simulink model "BLDCFramework"  (R2026a)
settings: Solver=FixedStepAuto  StopTime=4  FixedStep=6.25e-5
undefined symbols (not defined in the file): BldcControl_Params, BldcRuntime_Init
settings Model: DataDictionary=BldcData.sldd  Creator=k  LastModifiedBy=k
settings OptimizationCC: UseDivisionForNetSlopeComputation=on  GainParamInheritBuiltInType=on  UseFloatMulNetSlope=on  InlineInvariantSignals=on  NoFixptDivByZeroProtection=on  EfficientFloat2IntCast=on  LifeSpan=1
settings RTWCC: SystemTargetFile=ert.tlc  GenerateReport=on  Toolchain=MinGW64 | gmake (64-bit Windows)  IncludeHyperlinkInReport=on  GenerateTraceInfo=on  GenerateTraceReport=on  GenerateTraceReportSl=on  GenerateTraceReportSf=on  GenerateTraceReportEml=on  GenerateCodeMetricsReport=on  Description=Embedded Coder
settings ERTTargetCC: GenerateSampleERTMain=on  IncludeMdlTerminateFcn=off  CombineSignalStateStructs=on  SupportComplex=off  SupportContinuousTime=on  SupportNonInlinedSFcns=on

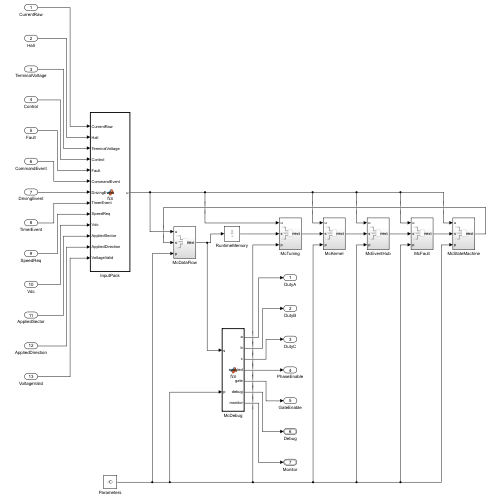
[thumbnail: Simulink's stored preview of the top-level diagram]
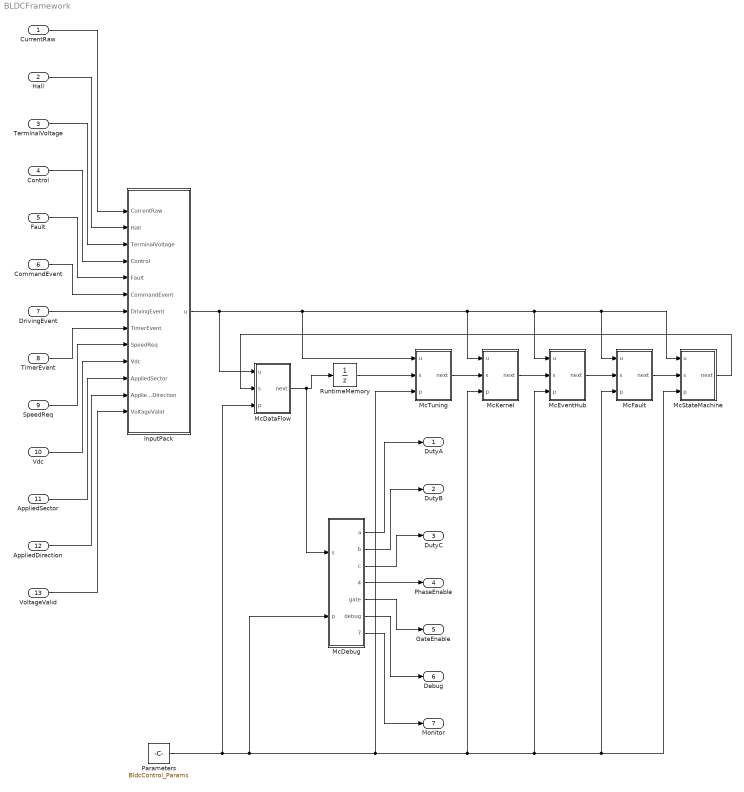
== system BLDCFramework ==
  CurrentRaw : Inport  OutDataTypeStr=uint16  PortDimensions=3  SampleTime=6.25e-5
  Hall : Inport  Port=2  OutDataTypeStr=uint8  PortDimensions=1  SampleTime=6.25e-5
  TerminalVoltage : Inport  Port=3  OutDataTypeStr=single  PortDimensions=3  SampleTime=6.25e-5
  Control : Inport  Port=4  OutDataTypeStr=uint8  PortDimensions=1  SampleTime=6.25e-5
  Fault : Inport  Port=5  OutDataTypeStr=boolean  PortDimensions=1  SampleTime=6.25e-5
  CommandEvent : Inport  Port=6  OutDataTypeStr=boolean  PortDimensions=1  SampleTime=6.25e-5
  DrivingEvent : Inport  Port=7  OutDataTypeStr=boolean  PortDimensions=1  SampleTime=6.25e-5
  TimerEvent : Inport  Port=8  OutDataTypeStr=boolean  PortDimensions=1  SampleTime=6.25e-5
  SpeedReq : Inport  Port=9  OutDataTypeStr=single  PortDimensions=1  SampleTime=6.25e-5
  Vdc : Inport  Port=10  OutDataTypeStr=single  PortDimensions=1  SampleTime=6.25e-5
  AppliedSector : Inport  Port=11  OutDataTypeStr=uint8  PortDimensions=1  SampleTime=6.25e-5
  AppliedDirection : Inport  Port=12  OutDataTypeStr=int8  PortDimensions=1  SampleTime=6.25e-5
  VoltageValid : Inport  Port=13  OutDataTypeStr=boolean  PortDimensions=1  SampleTime=6.25e-5
  InputPack : MATLAB Function  TreatAsAtomicUnit=on
  McDataFlow : Subsystem
  McDebug : MATLAB Function  TreatAsAtomicUnit=on
  McEventHub : Subsystem
  McFault : Subsystem
  McKernel : Subsystem
  McStateMachine : Subsystem
  McTuning : Subsystem
  Parameters : Constant  Value=BldcControl_Params  OutDataTypeStr=Bus: tBldcParams
  RuntimeMemory : UnitDelay  InitialCondition=BldcRuntime_Init  SampleTime=6.25e-5
  DutyA : Outport  OutDataTypeStr=uint16  PortDimensions=1
  DutyB : Outport  Port=2  OutDataTypeStr=uint16  PortDimensions=1
  DutyC : Outport  Port=3  OutDataTypeStr=uint16  PortDimensions=1
  PhaseEnable : Outport  Port=4  OutDataTypeStr=boolean  PortDimensions=3
  GateEnable : Outport  Port=5  OutDataTypeStr=boolean  PortDimensions=1
  Debug : Outport  Port=6  OutDataTypeStr=Bus: tBldcDebug  PortDimensions=1
  Monitor : Outport  Port=7  OutDataTypeStr=Bus: tBldcMonitor  PortDimensions=1
  wires:
  McDebug/7(monitor) -> Monitor/1
  McDebug/6(debug) -> Debug/1
  McDebug/5(gate) -> GateEnable/1
  McDebug/4(enabled) -> PhaseEnable/1
  McDebug/3(c) -> DutyC/1
  McDebug/2(b) -> DutyB/1
  McDebug/1(a) -> DutyA/1
  McDataFlow/1(next) -> McDebug/1(s), RuntimeMemory/1
  McStateMachine/1(next) -> McDataFlow/2(s)
  McFault/1(next) -> McStateMachine/2(s)
  McEventHub/1(next) -> McFault/2(s)
  McKernel/1(next) -> McEventHub/2(s)
  McTuning/1(next) -> McKernel/2(s)
  Parameters/1 -> McStateMachine/3(p), McFault/3(p), McEventHub/3(p), McKernel/3(p), McTuning/3(p), McDebug/2(p), McDataFlow/3(p)
  RuntimeMemory/1 -> McTuning/2(s)
  InputPack/1(u) -> McFault/1(u), McStateMachine/1(u), McEventHub/1(u), McKernel/1(u), McTuning/1(u), McDataFlow/1(u)
  VoltageValid/1 -> InputPack/13(VoltageValid)
  AppliedDirection/1 -> InputPack/12(AppliedDirection)
  AppliedSector/1 -> InputPack/11(AppliedSector)
  Vdc/1 -> InputPack/10(Vdc)
  SpeedReq/1 -> InputPack/9(SpeedReq)
  TimerEvent/1 -> InputPack/8(TimerEvent)
  DrivingEvent/1 -> InputPack/7(DrivingEvent)
  CommandEvent/1 -> InputPack/6(CommandEvent)
  Fault/1 -> InputPack/5(Fault)
  Control/1 -> InputPack/4(Control)
  TerminalVoltage/1 -> InputPack/3(TerminalVoltage)
  Hall/1 -> InputPack/2(Hall)
  CurrentRaw/1 -> InputPack/1(CurrentRaw)

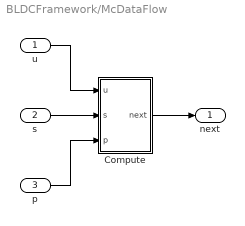
== system BLDCFramework/McDataFlow ==
  u : Inport  OutDataTypeStr=Bus: tBldcInput  PortDimensions=1  SampleTime=6.25e-5
  s : Inport  Port=2  OutDataTypeStr=Bus: tBldcRuntime  PortDimensions=1  SampleTime=6.25e-5
  p : Inport  Port=3  OutDataTypeStr=Bus: tBldcParams  PortDimensions=1  SampleTime=6.25e-5
  Compute : MATLAB Function  TreatAsAtomicUnit=on
  next : Outport  OutDataTypeStr=Bus: tBldcRuntime  PortDimensions=1
  wires:
  Compute/1(next) -> next/1
  p/1 -> Compute/3(p)
  s/1 -> Compute/2(s)
  u/1 -> Compute/1(u)

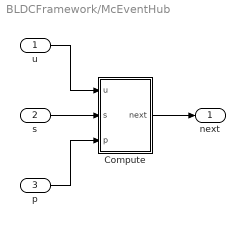
== system BLDCFramework/McEventHub ==
  u : Inport  OutDataTypeStr=Bus: tBldcInput  PortDimensions=1  SampleTime=6.25e-5
  s : Inport  Port=2  OutDataTypeStr=Bus: tBldcRuntime  PortDimensions=1  SampleTime=6.25e-5
  p : Inport  Port=3  OutDataTypeStr=Bus: tBldcParams  PortDimensions=1  SampleTime=6.25e-5
  Compute : MATLAB Function  TreatAsAtomicUnit=on
  next : Outport  OutDataTypeStr=Bus: tBldcRuntime  PortDimensions=1
  wires:
  Compute/1(next) -> next/1
  p/1 -> Compute/3(p)
  s/1 -> Compute/2(s)
  u/1 -> Compute/1(u)

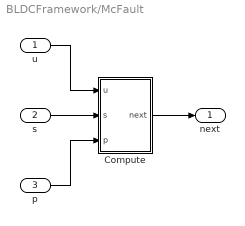
== system BLDCFramework/McFault ==
  u : Inport  OutDataTypeStr=Bus: tBldcInput  PortDimensions=1  SampleTime=6.25e-5
  s : Inport  Port=2  OutDataTypeStr=Bus: tBldcRuntime  PortDimensions=1  SampleTime=6.25e-5
  p : Inport  Port=3  OutDataTypeStr=Bus: tBldcParams  PortDimensions=1  SampleTime=6.25e-5
  Compute : MATLAB Function  TreatAsAtomicUnit=on
  next : Outport  OutDataTypeStr=Bus: tBldcRuntime  PortDimensions=1
  wires:
  Compute/1(next) -> next/1
  p/1 -> Compute/3(p)
  s/1 -> Compute/2(s)
  u/1 -> Compute/1(u)

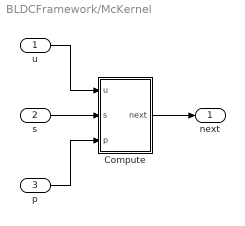
== system BLDCFramework/McKernel ==
  u : Inport  OutDataTypeStr=Bus: tBldcInput  PortDimensions=1  SampleTime=6.25e-5
  s : Inport  Port=2  OutDataTypeStr=Bus: tBldcRuntime  PortDimensions=1  SampleTime=6.25e-5
  p : Inport  Port=3  OutDataTypeStr=Bus: tBldcParams  PortDimensions=1  SampleTime=6.25e-5
  Compute : MATLAB Function  TreatAsAtomicUnit=on
  next : Outport  OutDataTypeStr=Bus: tBldcRuntime  PortDimensions=1
  wires:
  Compute/1(next) -> next/1
  p/1 -> Compute/3(p)
  s/1 -> Compute/2(s)
  u/1 -> Compute/1(u)

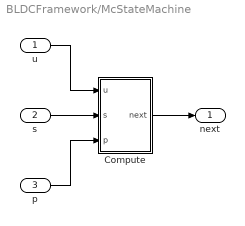
== system BLDCFramework/McStateMachine ==
  u : Inport  OutDataTypeStr=Bus: tBldcInput  PortDimensions=1  SampleTime=6.25e-5
  s : Inport  Port=2  OutDataTypeStr=Bus: tBldcRuntime  PortDimensions=1  SampleTime=6.25e-5
  p : Inport  Port=3  OutDataTypeStr=Bus: tBldcParams  PortDimensions=1  SampleTime=6.25e-5
  Compute : MATLAB Function  TreatAsAtomicUnit=on
  next : Outport  OutDataTypeStr=Bus: tBldcRuntime  PortDimensions=1
  wires:
  Compute/1(next) -> next/1
  p/1 -> Compute/3(p)
  s/1 -> Compute/2(s)
  u/1 -> Compute/1(u)

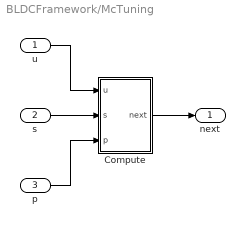
== system BLDCFramework/McTuning ==
  u : Inport  OutDataTypeStr=Bus: tBldcInput  PortDimensions=1  SampleTime=6.25e-5
  s : Inport  Port=2  OutDataTypeStr=Bus: tBldcRuntime  PortDimensions=1  SampleTime=6.25e-5
  p : Inport  Port=3  OutDataTypeStr=Bus: tBldcParams  PortDimensions=1  SampleTime=6.25e-5
  Compute : MATLAB Function  TreatAsAtomicUnit=on
  next : Outport  OutDataTypeStr=Bus: tBldcRuntime  PortDimensions=1
  wires:
  Compute/1(next) -> next/1
  p/1 -> Compute/3(p)
  s/1 -> Compute/2(s)
  u/1 -> Compute/1(u)

== matlab function BLDCFramework/McDebug ==
  data: s input; a output; p input; b output; c output; enabled output; gate output; debug output Bus: tBldcDebug; monitor output Bus: tBldcMonitor
function [a,b,c,enabled,gate,debug,monitor]=fcn(s,p)
%#codegen
[counts,enabled,gate,debug,monitor]=bldc.monitor(s,p);
a=counts(1);b=counts(2);c=counts(3);
end

== matlab function BLDCFramework/InputPack ==
  data: CurrentRaw input; u output Bus: tBldcInput; Hall input; TerminalVoltage input; Control input; Fault input; CommandEvent input; DrivingEvent input; TimerEvent input; SpeedReq input; Vdc input; AppliedSector input; AppliedDirection input; VoltageValid input
function u=fcn(CurrentRaw,Hall,TerminalVoltage,Control,Fault,CommandEvent,DrivingEvent,TimerEvent,SpeedReq,Vdc,AppliedSector,AppliedDirection,VoltageValid)
%#codegen
u.CurrentRaw=CurrentRaw;
u.Hall=Hall;
u.TerminalVoltage=TerminalVoltage;
u.Control=Control;
u.Fault=Fault;
u.CommandEvent=CommandEvent;
u.DrivingEvent=DrivingEvent;
u.TimerEvent=TimerEvent;
u.SpeedReq=SpeedReq;
u.Vdc=Vdc;
u.AppliedSector=AppliedSector;
u.AppliedDirection=AppliedDirection;
u.VoltageValid=VoltageValid;
end

== matlab function BLDCFramework/McTuning/Compute ==
  data: u input; next output Bus: tBldcRuntime; s input; p input
function next=fcn(u,s,p)
%#codegen
next=bldc.tuning(u,s,p);
end

== matlab function BLDCFramework/McKernel/Compute ==
  data: u input; next output Bus: tBldcRuntime; s input; p input
function next=fcn(u,s,p)
%#codegen
next=bldc.kernel(u,s,p);
end

== matlab function BLDCFramework/McEventHub/Compute ==
  data: u input; next output Bus: tBldcRuntime; s input; p input
function next=fcn(u,s,p)
%#codegen
next=bldc.event_hub(u,s,p);
end

== matlab function BLDCFramework/McFault/Compute ==
  data: u input; next output Bus: tBldcRuntime; s input; p input
function next=fcn(u,s,p)
%#codegen
next=bldc.protection(u,s,p);
end

== matlab function BLDCFramework/McStateMachine/Compute ==
  data: u input; next output Bus: tBldcRuntime; s input; p input
function next=fcn(u,s,p)
%#codegen
next=bldc.supervisor(u,s,p);
end

== matlab function BLDCFramework/McDataFlow/Compute ==
  data: u input; next output Bus: tBldcRuntime; s input; p input
function next=fcn(u,s,p)
%#codegen
next=bldc.dataflow(u,s,p);
end
